simulink library "mySTLLib"  (R2019b)
settings: Solver=ode45  StartTime=0.0  StopTime=10.0  RelTol=1e-3  EnableMultiTasking=on
libraries: simulink_extras x6, simulink x4
settings Model: Creator=balsi  LastModifiedBy=yuxia
settings DataIOCC: LimitDataPoints=on  SaveFormat=Array  ReturnWorkspaceOutputs=off
settings OptimizationCC: LifeSpan=inf
settings DebuggingCC: SFUnexpectedBacktrackingDiag=warning  SFNoUnconditionalDefaultTransitionDiag=warning  SFExecutionAtInitializationDiag=none  ArithmeticOperatorsInVariantConditions=warning
settings HardwareCC: ProdBitPerPointer=32  ProdBitPerSizeT=32  ProdBitPerPtrDiffT=32  ProdLargestAtomicFloat=None  ProdIntDivRoundTo=Undefined  ProdEndianess=Unspecified  ProdWordSize=32  ProdHWDeviceType=32-bit Generic
settings ModelReferenceCC: PropagateSignalLabelsOutOfModel=off
settings SFSimCC: SimUseLocalCustomCode=off  CustomCodeUndefinedFunction=UseInterfaceOnly
settings RTWCC: RTWUseLocalCustomCode=off
settings CodeAppCC: StateflowObjectComments=on
settings GRTTargetCC: TargetLangStandard=C89/C90 (ANSI)  GeneratePreprocessorConditionals=Disable all
settings ConfigComp: CovMetricSettings=dw  CovHtmlReporting=on  CovSaveCumulativeToWorkspaceVar=on  CovSaveSingleToWorkspaceVar=on  CovExternalEMLEnable=off

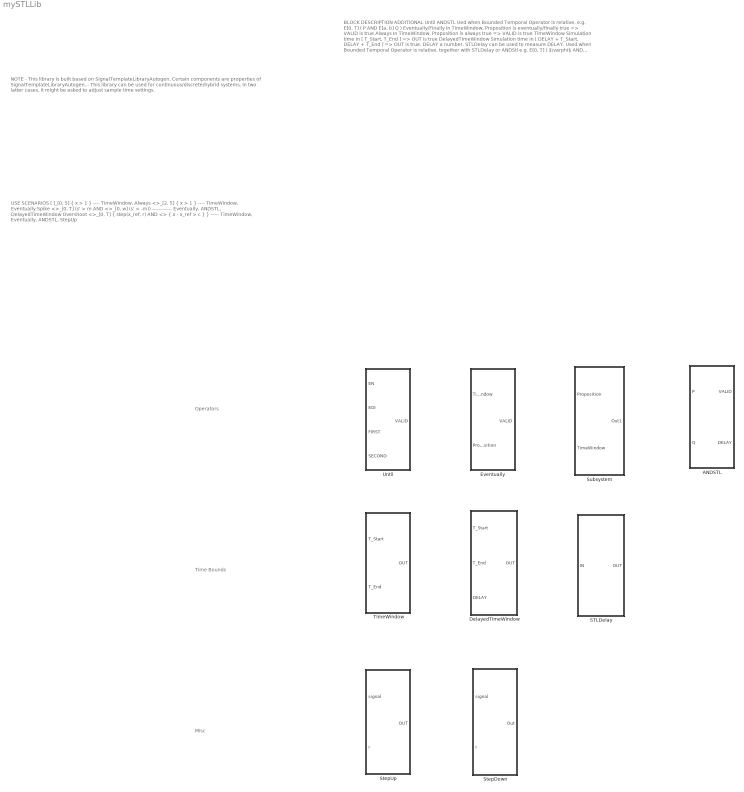
== system mySTLLib ==
  note: Operators
  note: USE SCENARIOS
      |
      | [ ]_[0, 5] { x > 1 } ---- TimeWindow, Always
      | <>_[2, 5] { x > 1 } ---- TimeWindow, Eventually
      | Spike <>_[0, T] (s' > m AND <>_[0, w] (s' < -m)) ------------ Eventually, ANDSTL, DelayedTimeWindow
      | Overshoot <>_[0, T] { step(x_ref, r) AND <> { x - x_ref > c } } ----- TimeWindow, Eventually, ANDSTL, StepUp
  note: BLOCK
      | DESCRIPTION
      | ADDITIONAL
      |
      | Until
      |
      | ANDSTL
      | Ued when Bounded Temporal Operator is relative,
      | e.g. E[0, T] ( P AND E[a, b] Q )
      |
      | Eventually/Finally
      | In TimeWindow, Proposition is eventually/finally true => VALID is true
      |
      | Always
      | In TimeWindow, Proposition is always true => VALID is true
      |
      | TimeWindow
      | Simulation time in [ T_Start, T_End ] => OUT is true
      |
      | DelayedTimeWindow
      | Simulation time in [ DELAY + T_Start, DELAY + T_End ] => OUT is true.
      | DELAY a number.
      | STLDelay can be used to measure DELAY.
      | Used when Bounded Temporal Operator is relative, together with STLDelay or ANDStl
      | e.g. E[0, T] ( $\varphi$ AND E[a, b] $\psi$ )
      |
      | STLDelay
      | Output reflects the time intant when input rises/falls sharply,
      |
      | e.g. a pulse arrives at t = 1.2 => OUT = 1.2
      | then a pulse leaves at t = 1.5 => OUT = 1.5
      | - Used when Bounded Temporal Operator is relative, together with DelayedTimeWindow.
      | - Output has a delay of $\epsilon$ , a parameter of Memory block inside. See block "Memory" for more info.
      |
      | Step(StepUp)
      | Step_Up Detector.
      | Detect the moment when signal(t + $\epsilon$ ) - signal(t) > r.
      | $\epsilon$ is delay.
      | It is a parameter of Memory block inside.
      | See block "Memory" for more info.
      |
      | StepDown
      | Step_Down Detector.
      | Detect the moment when - signal(t + $\epsilon$ ) + signal(t) > r.
      | $\epsilon$ is delay.
      | It is a parameter of Memory block inside.
      | See block "Memory" for more info.
  note: NOTE
      |
      | - This library is built based on SignalTemplateLibraryAutogen.
      | Certain components are properties of SignalTemplateLibraryAutogen.
      |
      | - This library can be used for continuous/discrete/hybrid systems.
      | In two latter cases, it might be asked to adjust sample time settings.
  note: Time Bounds
  note: Misc
  ANDSTL : Subsystem
  DelayedTimeWindow : Subsystem
  Eventually : Subsystem
  STLDelay : Subsystem
  StepDown : Subsystem
  StepUp : Subsystem
  Subsystem : Subsystem
  TimeWindow : Subsystem
  Until : Subsystem

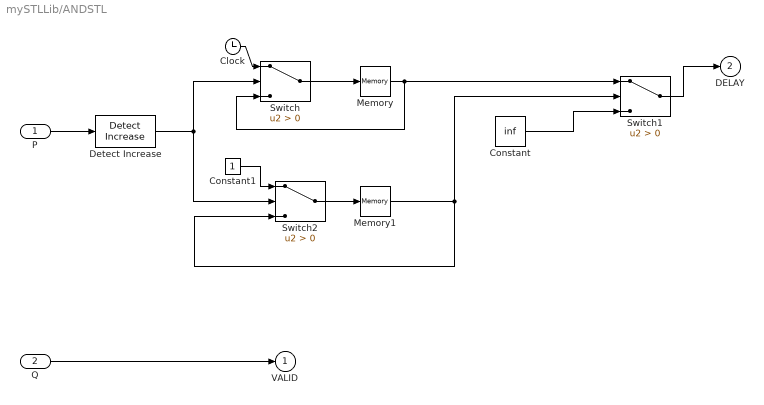
== system mySTLLib/ANDSTL ==
  P : Inport
  Q : Inport  Port=2
  Clock : Clock
  Constant : Constant  Value=inf
  Constant1 : Constant
  Detect Increase : simulink/Logic and Bit Operations/Detect Increase  vinit=0.0  OutDataTypeStr=boolean
  Memory : Memory
  Memory1 : Memory
  Switch : Switch  Criteria=u2 > Threshold
  Switch1 : Switch  Criteria=u2 > Threshold
  Switch2 : Switch  Criteria=u2 > Threshold
  VALID : Outport
  DELAY : Outport  Port=2
  wires:
  P/1 -> Detect Increase/1
  Q/1 -> VALID/1
  Memory/1 -> Switch1/1, Switch/3
  Memory1/1 -> Switch1/2, Switch2/3
  Switch/1 -> Memory/1
  Switch1/1 -> DELAY/1
  Constant/1 -> Switch1/3
  Switch2/1 -> Memory1/1
  Detect Increase/1 -> Switch/2, Switch2/2
  Constant1/1 -> Switch2/1
  Clock/1 -> Switch/1

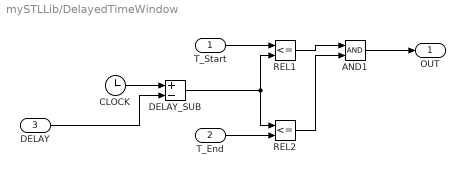
== system mySTLLib/DelayedTimeWindow ==
  T_Start : Inport
  T_End : Inport  Port=2
  DELAY : Inport  Port=3
  AND1 : Logic  AllPortsSameDT=off  OutDataTypeStr=boolean
  CLOCK : Clock
  DELAY_SUB : Sum  Inputs=+-
  REL1 : RelationalOperator  Operator=<=  OutDataTypeStr=boolean  RndMeth=Simplest
  REL2 : RelationalOperator  Operator=<=  OutDataTypeStr=boolean  RndMeth=Simplest
  OUT : Outport
  wires:
  REL1/1 -> AND1/1
  CLOCK/1 -> DELAY_SUB/1
  REL2/1 -> AND1/2
  T_Start/1 -> REL1/1
  DELAY_SUB/1 -> REL1/2, REL2/1
  AND1/1 -> OUT/1
  DELAY/1 -> DELAY_SUB/2
  T_End/1 -> REL2/2

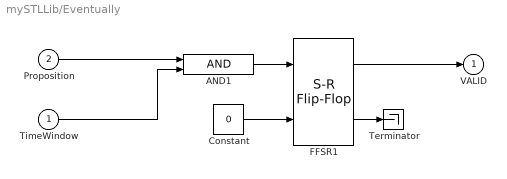
== system mySTLLib/Eventually ==
  TimeWindow : Inport
  Proposition : Inport  Port=2
  AND1 : Logic  AllPortsSameDT=off  OutDataTypeStr=boolean
  Constant : Constant  Value=0  OutDataTypeStr=boolean
  FFSR1 : simulink_extras/Flip Flops/S-R Flip-Flop  initial_condition=0
  Terminator : Terminator
  VALID : Outport
  wires:
  AND1/1 -> FFSR1/1
  FFSR1/2 -> Terminator/1
  Constant/1 -> FFSR1/2
  TimeWindow/1 -> AND1/2
  Proposition/1 -> AND1/1
  FFSR1/1 -> VALID/1

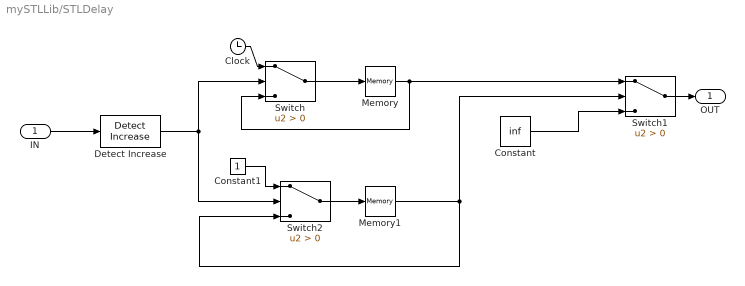
== system mySTLLib/STLDelay ==
  IN : Inport
  Clock : Clock
  Constant : Constant  Value=inf
  Constant1 : Constant
  Detect Increase : simulink/Logic and Bit Operations/Detect Increase  vinit=0.0  OutDataTypeStr=boolean
  Memory : Memory
  Memory1 : Memory
  Switch : Switch  Criteria=u2 > Threshold
  Switch1 : Switch  Criteria=u2 > Threshold
  Switch2 : Switch  Criteria=u2 > Threshold
  OUT : Outport
  wires:
  Clock/1 -> Switch/1
  Constant1/1 -> Switch2/1
  Memory1/1 -> Switch1/2, Switch2/3
  Switch/1 -> Memory/1
  Switch1/1 -> OUT/1
  Switch2/1 -> Memory1/1
  Detect Increase/1 -> Switch/2, Switch2/2
  IN/1 -> Detect Increase/1
  Memory/1 -> Switch1/1, Switch/3
  Constant/1 -> Switch1/3

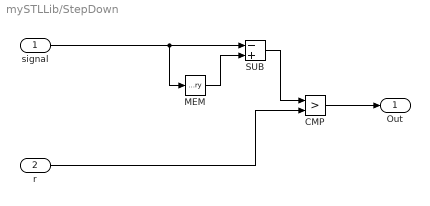
== system mySTLLib/StepDown ==
  signal : Inport
  r : Inport  Port=2
  CMP : RelationalOperator  Operator=>  OutDataTypeStr=boolean  RndMeth=Simplest
  MEM : Memory
  SUB : Sum  Inputs=-+
  Out : Outport
  wires:
  SUB/1 -> CMP/1
  signal/1 -> SUB/1, MEM/1
  MEM/1 -> SUB/2
  CMP/1 -> Out/1
  r/1 -> CMP/2

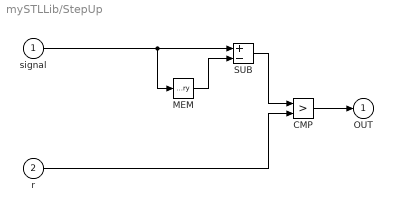
== system mySTLLib/StepUp ==
  signal : Inport
  r : Inport  Port=2
  CMP : RelationalOperator  Operator=>  OutDataTypeStr=boolean  RndMeth=Simplest
  MEM : Memory
  SUB : Sum  Inputs=+-
  OUT : Outport
  wires:
  MEM/1 -> SUB/2
  CMP/1 -> OUT/1
  signal/1 -> MEM/1, SUB/1
  SUB/1 -> CMP/1
  r/1 -> CMP/2

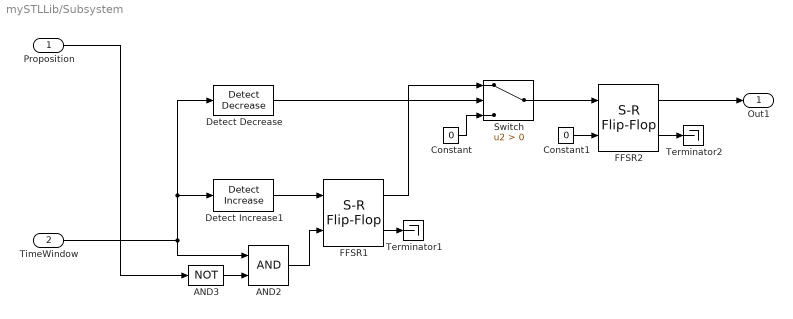
== system mySTLLib/Subsystem ==
  Proposition : Inport
  TimeWindow : Inport  Port=2
  AND2 : Logic  AllPortsSameDT=off  OutDataTypeStr=boolean
  AND3 : Logic  Operator=NOT  AllPortsSameDT=off  OutDataTypeStr=boolean
  Constant : Constant  Value=0  OutDataTypeStr=boolean
  Constant1 : Constant  Value=0  OutDataTypeStr=boolean
  Detect Decrease : simulink/Logic and Bit Operations/Detect Decrease  vinit=0.0  OutDataTypeStr=boolean
  Detect Increase1 : simulink/Logic and Bit Operations/Detect Increase  vinit=0.0  OutDataTypeStr=boolean
  FFSR1 : simulink_extras/Flip Flops/S-R Flip-Flop  initial_condition=0
  FFSR2 : simulink_extras/Flip Flops/S-R Flip-Flop  initial_condition=0
  Switch : Switch  Criteria=u2 > Threshold
  Terminator1 : Terminator
  Terminator2 : Terminator
  Out1 : Outport
  wires:
  Switch/1 -> FFSR2/1
  Constant1/1 -> FFSR2/2
  Constant/1 -> Switch/3
  Detect Decrease/1 -> Switch/2
  Proposition/1 -> AND3/1
  AND2/1 -> FFSR1/2
  FFSR2/2 -> Terminator2/1
  FFSR2/1 -> Out1/1
  AND3/1 -> AND2/2
  TimeWindow/1 -> Detect Decrease/1, Detect Increase1/1, AND2/1
  Detect Increase1/1 -> FFSR1/1
  FFSR1/1 -> Switch/1
  FFSR1/2 -> Terminator1/1

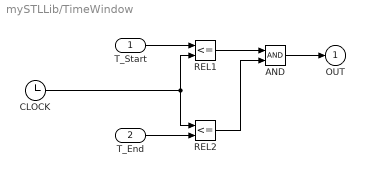
== system mySTLLib/TimeWindow ==
  T_Start : Inport
  T_End : Inport  Port=2
  AND : Logic  AllPortsSameDT=off  OutDataTypeStr=boolean
  CLOCK : Clock
  REL1 : RelationalOperator  Operator=<=  OutDataTypeStr=boolean  RndMeth=Simplest
  REL2 : RelationalOperator  Operator=<=  OutDataTypeStr=boolean  RndMeth=Simplest
  OUT : Outport
  wires:
  CLOCK/1 -> REL1/2, REL2/1
  T_End/1 -> REL2/2
  REL1/1 -> AND/1
  REL2/1 -> AND/2
  AND/1 -> OUT/1
  T_Start/1 -> REL1/1

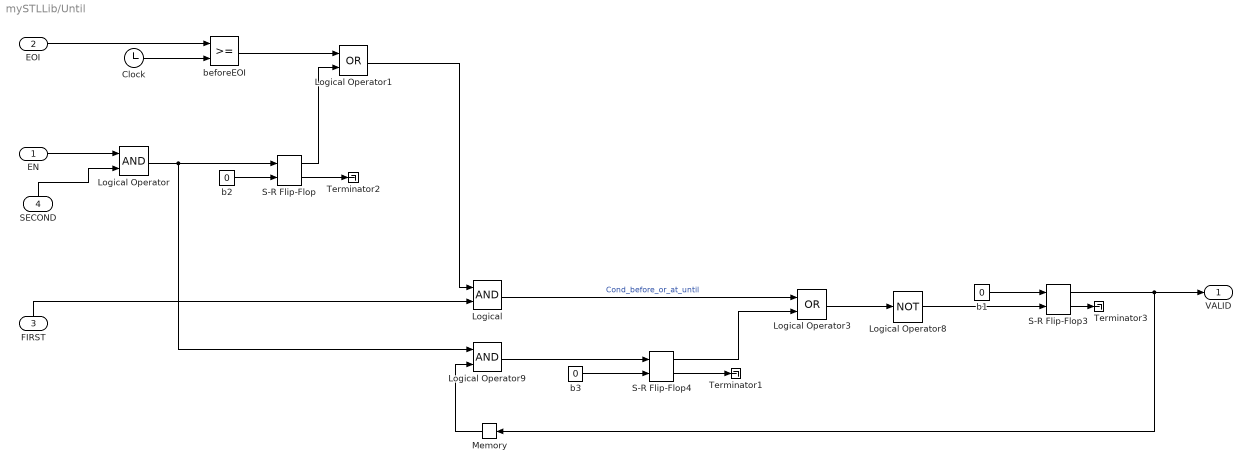
== system mySTLLib/Until ==
  EN : Inport
  EOI : Inport  Port=2
  FIRST : Inport  Port=3
  SECOND : Inport  Port=4
  Clock : Clock
  "Logical " : Logic  AllPortsSameDT=off  OutDataTypeStr=boolean
  Logical Operator : Logic  AllPortsSameDT=off  OutDataTypeStr=boolean
  Logical Operator1 : Logic  Operator=OR  AllPortsSameDT=off  OutDataTypeStr=boolean
  Logical Operator3 : Logic  Operator=OR  AllPortsSameDT=off  OutDataTypeStr=boolean
  Logical Operator8 : Logic  Operator=NOT  Inputs=1  AllPortsSameDT=off  OutDataTypeStr=boolean
  Logical Operator9 : Logic  AllPortsSameDT=off  OutDataTypeStr=boolean
  Memory : Memory
  S-R Flip-Flop : simulink_extras/Flip Flops/S-R Flip-Flop  initial_condition=0
  S-R Flip-Flop3 : simulink_extras/Flip Flops/S-R Flip-Flop  initial_condition=1
  S-R Flip-Flop4 : simulink_extras/Flip Flops/S-R Flip-Flop  initial_condition=0
  Terminator1 : Terminator
  Terminator2 : Terminator
  Terminator3 : Terminator
  b1 : Constant  Value=0  OutDataTypeStr=boolean
  b2 : Constant  Value=0  OutDataTypeStr=boolean
  b3 : Constant  Value=0  OutDataTypeStr=boolean
  beforeEOI : RelationalOperator  OutDataTypeStr=boolean  RndMeth=Nearest
  VALID : Outport
  wires:
  S-R Flip-Flop/2 -> Terminator2/1
  "Logical "/1 -> Logical Operator3/1  "Cond_before_or_at_until"
  S-R Flip-Flop4/2 -> Terminator1/1
  Clock/1 -> beforeEOI/2
  b1/1 -> S-R Flip-Flop3/1
  S-R Flip-Flop3/2 -> Terminator3/1
  EN/1 -> Logical Operator/1
  b2/1 -> S-R Flip-Flop/2
  Logical Operator1/1 -> "Logical "/1
  Logical Operator/1 -> S-R Flip-Flop/1, Logical Operator9/1
  S-R Flip-Flop3/1 -> VALID/1, Memory/1
  beforeEOI/1 -> Logical Operator1/1
  Logical Operator3/1 -> Logical Operator8/1
  SECOND/1 -> Logical Operator/2
  FIRST/1 -> "Logical "/2
  Memory/1 -> Logical Operator9/2
  Logical Operator9/1 -> S-R Flip-Flop4/1
  S-R Flip-Flop/1 -> Logical Operator1/2
  S-R Flip-Flop4/1 -> Logical Operator3/2
  Logical Operator8/1 -> S-R Flip-Flop3/2
  EOI/1 -> beforeEOI/1
  b3/1 -> S-R Flip-Flop4/2
